simulink model "rocket_sim_mpc"  (R2023a)
settings: Solver=ode45  StartTime=0.0  StopTime=20.0  MaxStep=0.01  RelTol=1e-3  EnableMultiTasking=on
libraries: simulink_extras x4, simulink x2, sharedtransform x2, shared6dof x1, aerolibanim x1, matrix_library x1
settings Model: Creator=jgillis  LastModifiedBy=aneki
settings SolverCC: AlgebraicLoopSolver=TrustRegion
settings DataIOCC: LimitDataPoints=on  SaveFormat=Array  ReturnWorkspaceOutputs=off
settings OptimizationCC: LifeSpan=inf
settings DebuggingCC: SolverPrmCheckMsg=warning  UnconnectedInputMsg=warning  UnconnectedOutputMsg=warning  UnconnectedLineMsg=warning  SFUnexpectedBacktrackingDiag=warning  SFNoUnconditionalDefaultTransitionDiag=warning  SFExecutionAtInitializationDiag=none  ArithmeticOperatorsInVariantConditions=warning
settings HardwareCC: ProdBitPerPointer=32  ProdBitPerSizeT=32  ProdBitPerPtrDiffT=32  ProdLargestAtomicFloat=None  ProdIntDivRoundTo=Undefined  ProdEndianess=Unspecified  ProdWordSize=32  ProdHWDeviceType=32-bit Generic
settings ModelReferenceCC: PropagateSignalLabelsOutOfModel=off
settings SFSimCC: SimUseLocalCustomCode=off  CustomCodeUndefinedFunction=UseInterfaceOnly
settings RTWCC: RTWUseLocalCustomCode=off
settings CodeAppCC: StateflowObjectComments=on
settings GRTTargetCC: TargetLangStandard=C89/C90 (ANSI)
settings ConfigComp: CovMetricSettings=dw  CovSaveCumulativeToWorkspaceVar=on  CovSaveSingleToWorkspaceVar=on  CovExternalEMLEnable=off  CovSFcnEnable=off

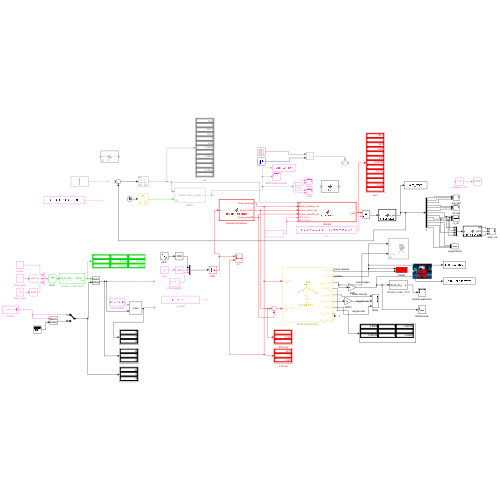
[thumbnail: Simulink's stored preview of the top-level diagram]
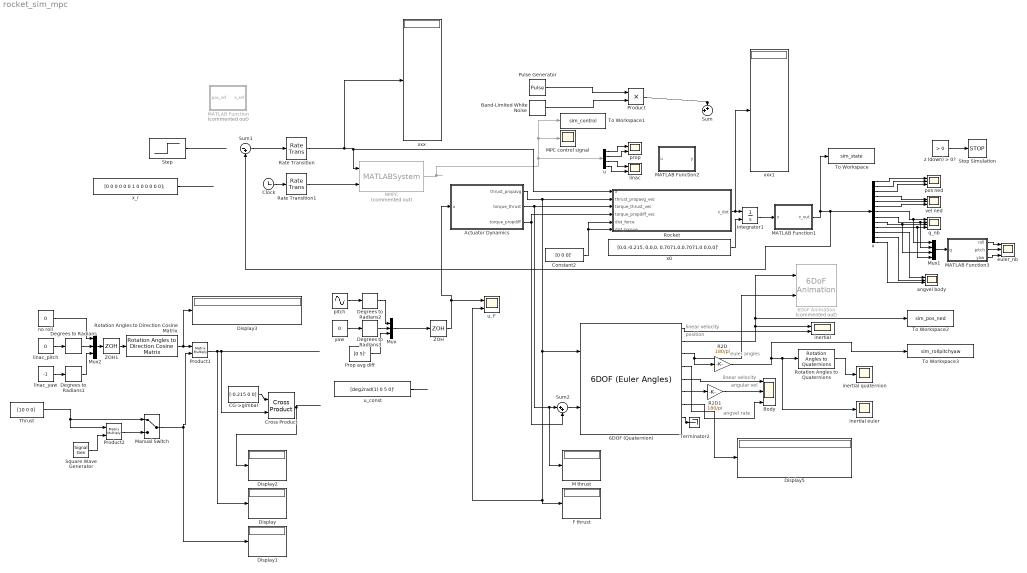
== system rocket_sim_mpc ==
  note: angvel rate
  note: linear velocity
  note: angular vel
  note: euler angles
  note: linear velocity
  note: position
  6DOF (Quaternion) : shared6dof/6DOF (Euler Angles)  units=Metric (MKS)  mtype=Fixed  rep=Quaternion  xme_0=[0 0 0.215]  Vm_0=[0 0 0]  eul_0=[0 0 0]  pm_0=[0 0 0]  mass_0=1.67  mass_e=0.5  mass_f=2.0  inertia=diag([0.0128, 0.0644, 0.0644])  inertia_e=eye(3)  inertia_f=2*eye(3)  k_quat=1  vre_flag=on  abi_flag=on  aMode=0  xme_statename={'x', 'y', 'z'}  Vm_statename={'vel_x', 'vel_y', 'vel_z'}  eul_statename=''  quat_statename={'qw', 'qx', 'qy', 'qz'}  pm_statename={'angvel_x', 'angvel_y', 'angvel_z'}  mass_statename=''
      settings: LibrarySourceBlock=aerolib6dof2/6DOF (Quaternion)
  6DoF Animation : aerolibanim/6DoF Animation  Commented=on  u1=[-2000 2000 -2000 2000 -2000 0]  u2=0.1  u3=5.0  u4=[4000 0 -5000]  u5=Fixed position  u6=[2000 500 -3150]  u7=10  u8=on
  Actuator Dynamics : MATLAB Function  TreatAsAtomicUnit=on
  Band-Limited White Noise : simulink/Sources/Band-Limited White Noise  Cov=[1]  Ts=10  seed=[23341]
  Body : Scope  NumInputPorts=3
  CG->gimbal : Constant  Value=[-0.215 0 0]
  Clock : Clock
  Constant2 : Constant  Value=[0 0 0]'
  Cross Product : matrix_library/Cross Product
  Degrees to Radians{,1..3} (4 alike) : simulink_extras/Transformations/Degrees to Radians
  Display{,1..3,5} (5 alike) : Display
  F thrust : Display
  Integrator1 : Integrator  InitialConditionSource=external
  M thrust : Display
  MATLAB Function : MATLAB Function  Commented=on  TreatAsAtomicUnit=on
  MATLAB Function1 : MATLAB Function  TreatAsAtomicUnit=on
  MATLAB Function2 : MATLAB Function  TreatAsAtomicUnit=on
  MATLAB Function3 : MATLAB Function  TreatAsAtomicUnit=on
  MPC control signal : Scope
  Manual Switch : ManualSwitch
  Mux : Mux  Inputs=3
  Mux1 : Mux
  Mux2 : Mux  Inputs=3
  NMPC : MATLABSystem  Commented=on  System=casadi_block_rocket  SimulateUsing=Interpreted execution
      mask Type: casadi_block_rocket
      mask Display:
      | disp('casadi_block_rocket');
      | port_label('output',1,'u');
  Product : Product
  Product1 : Product  Multiplication=Matrix(*)
  Product2 : Product  Multiplication=Matrix(*)
  Prop avg diff : Constant  Value=[0 5]'
  Pulse Generator : DiscretePulseGenerator  PulseType=Time based  Period=10  PulseWidth=5  PhaseDelay=10
  R2D : Gain  Gain=180/pi
  R2D1 : Gain  Gain=180/pi
  Rate Transition : RateTransition  InitialCondition=[0,0,-0.215, 0,0,0, 0.7071,0,0.7071,0 0,0,0]'  OutPortSampleTimeOpt=Inherit  OutPortSampleTime=0.5
  Rate Transition1 : RateTransition  OutPortSampleTime=0.5
  Rocket : MATLAB Function  TreatAsAtomicUnit=on
      settings: MinAlgLoopOccurrences=on
  Rotation Angles to Direction Cosine Matrix : sharedtransform/Rotation Angles to Direction Cosine Matrix  rotationOrder=ZYX  aMode=aMode
  Rotation Angles to Quaternions : sharedtransform/Rotation Angles to Quaternions  rotationOrder=ZYX  aMode=aMode
  Square Wave Generator : SignalGenerator  WaveForm=square  Frequency=0.5  Units=rad/sec
  Step : Step  Before=[0, 0, 10, 0, 0, 0, 1, 0, 0, 0, 0, 0, 0]'  After=[0, 0, 0, 0, 0, 0, 1, 0, 0, 0, 0, 0, 0]'  SampleTime=0
  Stop Simulation : Stop
  Sum : Sum  Inputs=++|
  Sum1 : Sum  Inputs=|-+
  Sum2 : Sum  Inputs=|++
  Terminator2 : Terminator
  Thrust : Constant  Value=[10 0 0]
  To Workspace : ToWorkspace  VariableName=sim_state  SaveFormat=Structure With Time  SampleTime=-1
  To Workspace1 : ToWorkspace  VariableName=sim_control  SaveFormat=Structure With Time  SampleTime=-1
  To Workspace2 : ToWorkspace  VariableName=sim_pos_ned  SaveFormat=Structure With Time  SampleTime=-1
  To Workspace3 : ToWorkspace  VariableName=sim_rollpitchyaw  SaveFormat=Structure With Time  SampleTime=-1
  ZOH : ZeroOrderHold  SampleTime=0.25
  ZOH1 : ZeroOrderHold  SampleTime=0.5
  angvel body : Scope  NumInputPorts=3
  euler_nb : Scope  NumInputPorts=3
  inertial : Scope  NumInputPorts=2
  inertial euler : Scope
  inertial quaternion : Scope
  linac : Scope  NumInputPorts=2
  linac_pitch : Constant  Value=0
  linac_yaw : Constant  Value=-1
  no roll : Constant  Value=0
  pitch : Sin  Amplitude=10  Phase=-pi/2  SampleTime=0
  pos ned : Scope  NumInputPorts=3
  prop : Scope  NumInputPorts=2
  q_nb : Scope  NumInputPorts=4
  u : Demux
  "u, F" : Scope  NumInputPorts=2
  u_const : Constant  Value=[deg2rad(1) 0 5 0]'  VectorParams1D=off
  vel ned : Scope  NumInputPorts=3
  x : Demux  Outputs=13
  x0 : Constant  Value=[0,0,-0.215, 0,0,0, 0.7071,0,0.7071,0 0,0,0]'  LockScale=on
  x_r : Constant  Value=[0 0 0 0 0 0 1 0 0 0 0 0 0];
  xxx : Display
  xxx1 : Display
  yaw : Constant  Value=0
  z (down) > 0? : simulink/Logic and Bit Operations/Compare To Constant  relop=>  const=0  OutDataTypeStr=boolean
  wires:
  NMPC/1 -> u/1, MPC control signal/1, To Workspace1/1
  Clock/1 -> Rate Transition1/1
  Rate Transition/1 -> xxx/1, Rocket/1(x), NMPC/1
  Band-Limited White Noise/1 -> Product/2
  Product/1 -> Sum/1
  Pulse Generator/1 -> Product/1
  ZOH/1 -> "u, F"/1, Actuator Dynamics/1(u)
  Rocket/1(x_dot) -> xxx1/1, Integrator1/1
  Constant2/1 -> Rocket/5(dist_force), Rocket/6(dist_torque)
  x/4 -> vel ned/1
  x/6 -> vel ned/3
  x/7 -> q_nb/1, Mux1/1
  x/8 -> q_nb/2, Mux1/2
  x/9 -> q_nb/3, Mux1/3
  x/10 -> Mux1/4, q_nb/4
  x/5 -> vel ned/2
  x/1 -> pos ned/1
  x/2 -> pos ned/2
  x/3 -> pos ned/3
  x/11 -> angvel body/1
  x/12 -> angvel body/2
  x/13 -> angvel body/3
  u/1 -> prop/1
  u/2 -> prop/2
  u/3 -> linac/1
  u/4 -> linac/2
  x_r/1 -> ?
  Step/1 -> ?
  Sum1/1 -> Rate Transition/1
  u_const/1 -> ?
  x0/1 -> Integrator1/2
  Product1/1 -> Display/1, Cross Product/2
  linac_pitch/1 -> Degrees to Radians/1
  linac_yaw/1 -> Degrees to Radians1/1
  Degrees to Radians1/1 -> Mux2/3
  Degrees to Radians/1 -> Mux2/2
  no roll/1 -> Mux2/1
  Mux2/1 -> ZOH1/1
  Rotation Angles to Direction Cosine Matrix/1 -> Display3/1, Product1/1
  Thrust/1 -> Manual Switch/1, Product2/1
  CG->gimbal/1 -> Cross Product/1
  Cross Product/1 -> Display2/1
  6DOF (Quaternion)/1 -> inertial/2
  6DOF (Quaternion)/2 -> To Workspace2/1, 6DoF Animation/1, inertial/1
  6DOF (Quaternion)/3 -> R2D/1, 6DoF Animation/2
  R2D/1 -> To Workspace3/1, inertial euler/1, Rotation Angles to Quaternions/1
  6DOF (Quaternion)/5 -> Body/1
  6DOF (Quaternion)/6 -> R2D1/1
  R2D1/1 -> Body/2
  6DOF (Quaternion)/7 -> Body/3
  6DOF (Quaternion)/8 -> Terminator2/1
  6DOF (Quaternion)/4 -> Display5/1
  Square Wave Generator/1 -> Product2/2
  Product2/1 -> Manual Switch/2
  Manual Switch/1 -> Display1/1, Product1/2
  Rotation Angles to Quaternions/1 -> inertial quaternion/1
  ZOH1/1 -> Rotation Angles to Direction Cosine Matrix/1
  Actuator Dynamics/1(thrust_propavg) -> 6DOF (Quaternion)/1, F thrust/1, "u, F"/2, Rocket/2(thrust_propavg_vec)
  Actuator Dynamics/2(torque_thrust) -> M thrust/1, Sum2/1, Rocket/3(torque_thrust_vec)
  Actuator Dynamics/3(torque_propdiff) -> Sum2/2, Rocket/4(torque_propdiff_vec)
  Sum2/1 -> 6DOF (Quaternion)/2
  Rate Transition1/1 -> NMPC/2
  Prop avg diff/1 -> Mux/3
  pitch/1 -> Degrees to Radians2/1
  Mux/1 -> ZOH/1
  yaw/1 -> Degrees to Radians3/1
  z (down) > 0?/1 -> Stop Simulation/1
  Degrees to Radians2/1 -> Mux/1
  Degrees to Radians3/1 -> Mux/2
  Integrator1/1 -> MATLAB Function1/1(x)
  MATLAB Function1/1(x_out) -> Sum1/2, x/1, To Workspace/1
  Mux1/1 -> MATLAB Function3/1(q)
  MATLAB Function3/1(roll) -> euler_nb/1
  MATLAB Function3/2(pitch) -> euler_nb/2
  MATLAB Function3/3(yaw) -> euler_nb/3

== matlab function rocket_sim_mpc/Actuator Dynamics ==
  data: u input; thrust_propavg output; torque_thrust output; torque_propdiff output
function [thrust_propavg, torque_thrust, torque_propdiff] = actuator_dynamics(u)
    [thrust_propavg, torque_thrust, torque_propdiff] = actuator_dynamics_f(u);
end

== matlab function rocket_sim_mpc/MATLAB Function ==
  data: pos_ref input; x_ref output
function x_ref = fcn(pos_ref)
% reference generator
y = u;

== matlab function rocket_sim_mpc/Rocket ==
  data: x input; thrust_propavg_vec input; torque_thrust_vec input; torque_propdiff_vec input; x_dot output; dist_force input; dist_torque input
function x_dot = rocket_model(x, thrust_propavg_vec, torque_thrust_vec, torque_propdiff_vec, dist_force, dist_torque)
    x_dot = rocket_model_f(x, thrust_propavg_vec, torque_thrust_vec, torque_propdiff_vec, dist_force, dist_torque);
end

== matlab function rocket_sim_mpc/MATLAB Function1 ==
  data: x input; x_out output
function x_out = q_normalize(x)
    q = x(7:10);
    if q(1) < 0 % handling quaternion ambiguity
        q = -q;
    end
    x(7:10) = q / norm(q);
    x_out = x;

end

== matlab function rocket_sim_mpc/MATLAB Function2 ==
  data: u input; y output
function y = fcn(u)

y = u;

== matlab function rocket_sim_mpc/MATLAB Function3 ==
  data: q input; roll output; pitch output; yaw output
function [roll,pitch,yaw] = q_to_euler_deg(q)
    [roll, pitch,yaw] = q2euler(q);
    roll = rad2deg(roll); pitch = deg2rad(pitch); yaw = deg2rad(yaw);
end
